simulink model "Exercise_3"  (R2024b)
settings: Solver=VariableStepAuto  StartTime=0.0  StopTime=10.0  RelTol=1e-3
settings Model: Creator=HP  LastModifiedBy=HP

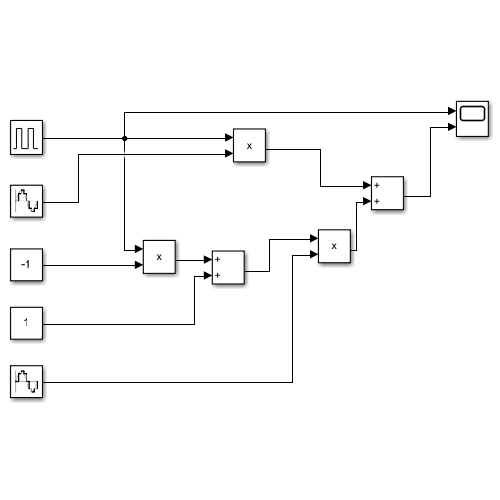
[thumbnail: Simulink's stored preview of the top-level diagram]
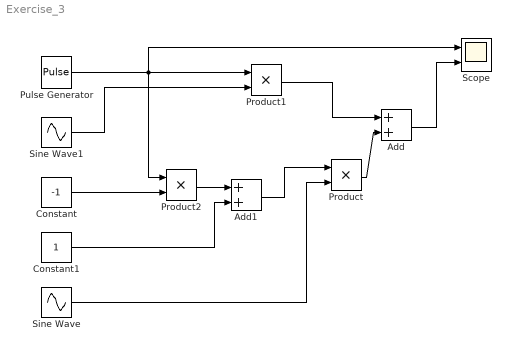
== system Exercise_3 ==
  Add : Sum
  Add1 : Sum
  Constant : Constant  Value=-1
  Constant1 : Constant
  Product : Product
  Product1 : Product
  Product2 : Product
  Pulse Generator : DiscretePulseGenerator  PulseType=Time based  PulseWidth=50
  Scope : Scope  NumInputPorts=2
  Sine Wave : Sin  Frequency=200  SampleTime=0.0001
  Sine Wave1 : Sin  Frequency=20  SampleTime=0.0001
  wires:
  Pulse Generator/1 -> Product2/1, Scope/1, Product1/1
  Product1/1 -> Add/1
  Product/1 -> Add/2
  Sine Wave/1 -> Product/2
  Sine Wave1/1 -> Product1/2
  Product2/1 -> Add1/1
  Constant/1 -> Product2/2
  Constant1/1 -> Add1/2
  Add1/1 -> Product/1
  Add/1 -> Scope/2
